simulink model "SintegrativeSP"  (R2022b)
settings: Solver=VariableStepAuto  StartTime=0.0  StopTime=Tsim  RelTol=1e-3
values from neighbouring files (symbols this model uses):
  Ampdist = -0.05    [integrative.m]
  Tdist = 75    [integrative.m]
  Tinit = 10    [integrative.m]
libraries: cstblocks x4, simulink x1
settings Model: Creator=jprmj  LastModifiedBy=jprmj

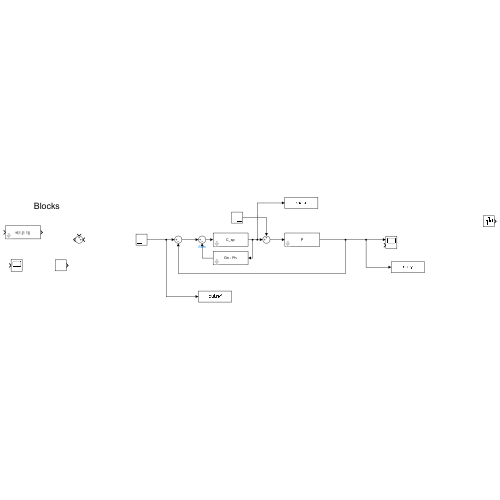
[thumbnail: Simulink's stored preview of the top-level diagram]
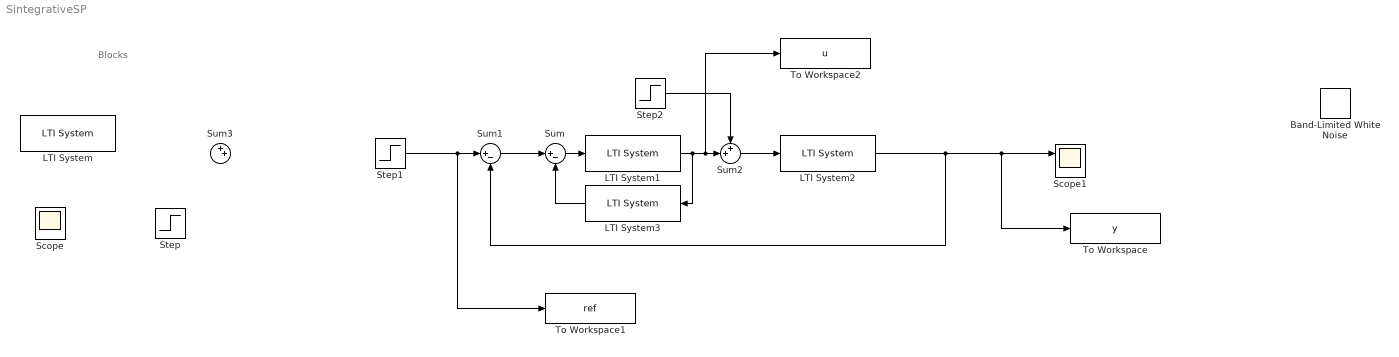
== system SintegrativeSP ==
  note: Blocks
  Band-Limited White Noise : simulink/Sources/Band-Limited White Noise  Cov=[0.1]  Ts=0.1  seed=[23341]
  LTI System : cstblocks/LTI System  sys=tf(1,[1 1])  IC=[]
  LTI System1 : cstblocks/LTI System  sys=C_sp  IC=[]
  LTI System2 : cstblocks/LTI System  sys=P  IC=[]
  LTI System3 : cstblocks/LTI System  sys=Gn - Pn  IC=[]
  Scope : Scope
  Scope1 : Scope  NumInputPorts=2
  Step : Step  SampleTime=0
  Step1 : Step  SampleTime=Tinit
  Step2 : Step  After=Ampdist  SampleTime=Tdist
  Sum : Sum  Inputs=|+-
  Sum1 : Sum  Inputs=|+-
  Sum2 : Sum  Inputs=++|
  Sum3 : Sum  Inputs=++|
  To Workspace : ToWorkspace  VariableName=y  SaveFormat=Timeseries  SampleTime=-1
  To Workspace1 : ToWorkspace  VariableName=ref  SaveFormat=Timeseries  SampleTime=-1
  To Workspace2 : ToWorkspace  VariableName=u  SaveFormat=Timeseries  SampleTime=-1
  wires:
  Step1/1 -> To Workspace1/1, Sum1/1
  Sum2/1 -> LTI System2/1
  LTI System1/1 -> LTI System3/1, To Workspace2/1, Sum2/2
  LTI System2/1 -> Sum1/2, To Workspace/1, Scope1/1
  Step2/1 -> Sum2/1
  Sum1/1 -> Sum/1
  Sum/1 -> LTI System1/1
  LTI System3/1 -> Sum/2
